simulink model "lab41"  (Simulink 8.0)
settings: Solver=ode45  StartTime=0.0  StopTime=10.0  RelTol=1e-3
undefined symbols (not defined in the file): get
libraries: commsequence2 x1, commseqgen2 x1, dspspect3 x1, simulink x1, commutil2 x1, dspsnks4 x1
settings Model: Creator=Dimav  LastModifiedBy=Dimav

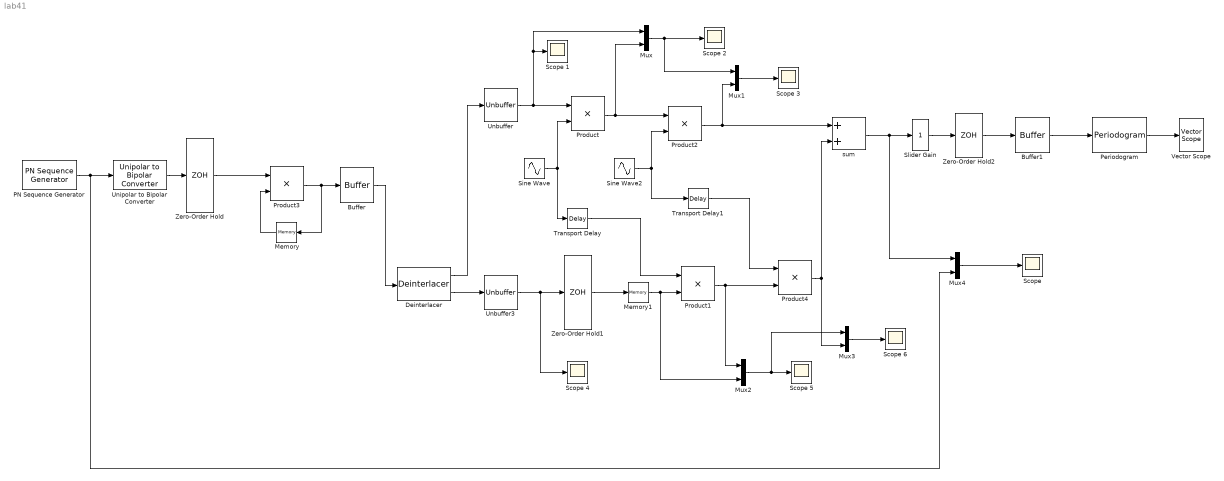
== system lab41 ==
  Buffer : Buffer  N=2  TreatMby1Signals=One channel
  Buffer1 : Buffer  TreatMby1Signals=One channel
  Deinterlacer : commsequence2/Deinterlacer
  Memory : Memory  X0=1  InheritSampleTime=on
  Memory1 : Memory  InheritSampleTime=on
  Mux{,1..4} (5 alike) : Mux  Inputs=2
  PN Sequence Generator : commseqgen2/PN Sequence Generator  poly=[1 0 0 0 0 1 1]  ini_sta=[0 0 0 0 0 1]  outBitMaskSource=Dialog parameter  shift=0  outVarSiz=off  maxOutSizeMode=Dialog parameter  maxOutSize=[10 1]  Ts=1/1200  frameBased=off  sampPerFrame=1  reset=off  bitPackedOutputs=off  outDataType=double  numPackedBits=8  bitPackDataSigned=off  bitPackedOutDType=double
  Periodogram : dspspect3/Periodogram  measurement=Power spectral density  wintype=Hamming  Rs=50  beta=5  winsamp=Symmetric  FFTImplementation=Auto  inheritFFT=off  fftsize=256  navg=4  inheritTs=on  Ts=1
  Product{,1..4} (5 alike) : Product  RndMeth=Zero
  Scope : Scope
      settings: SaveName=ScopeData6
  Scope {1..6} (6 alike) : Scope
      Scope 2 settings: SaveName=ScopeData2
      Scope 3 settings: SaveName=ScopeData3
      Scope 5 settings: SaveName=ScopeData4
      Scope 6 settings: SaveName=ScopeData5
  Sine Wave : Sin  Frequency=600*pi  Phase=-pi  SampleTime=0
  Sine Wave2 : Sin  Frequency=76000*pi  SampleTime=0
  Slider Gain : simulink/Math Operations/Slider Gain  low=0  gain=1  high=2
  Transport Delay : TransportDelay  DelayTime=1/1200
  Transport Delay1 : TransportDelay  DelayTime=3/38000/4
  Unbuffer : Unbuffer  SampleBasedProcessing=Same as frame based
  Unbuffer3 : Unbuffer  SampleBasedProcessing=Same as frame based
  Unipolar to Bipolar Converter : commutil2/Unipolar to Bipolar Converter  M=2  polarity=Positive  dataType=Inherit via internal rule
  Vector Scope : dspsnks4/Vector Scope  ScopeProperties=on  Domain=Time  HorizSpan=1  DisplayProperties=off  AxisGrid=on  Memory=off  FrameNumber=on  AxisLegend=off  AxisZoom=off  OpenScopeAtSimStart=on  OpenScopeImmediately=off  FigPos=get(0,'defaultfigureposition')  AxisProperties=off  XUnits=Hertz  XRange=[0...Fs/2]  InheritXIncr=on  XIncr=1  XLabel=Time  XLimit=Auto  XMin=0  XMax=1  XStart=0  YUnits=dB  YLabel=Amplitude  LineProperties=off  XAxisParamsVer=6.9
      settings: YMin=-10  YMax=10
  Zero-Order Hold : ZeroOrderHold  SampleTime=1/1200
  Zero-Order Hold1 : ZeroOrderHold  SampleTime=1/1200
  Zero-Order Hold2 : ZeroOrderHold  SampleTime=1/4000/3
  sum : Sum  Inputs=2  SaturateOnIntegerOverflow=on  InputSameDT=on  OutDataTypeStr=Inherit: Same as first input
  wires:
  Unipolar to Bipolar Converter/1 -> Zero-Order Hold/1
  Zero-Order Hold/1 -> Product3/1
  Memory/1 -> Product3/2
  Product3/1 -> Memory/1, Buffer/1
  Buffer/1 -> Deinterlacer/1
  Unbuffer/1 -> Mux/1, Scope 1/1, Product/1
  Sine Wave/1 -> Transport Delay/1, Product/2
  Unbuffer3/1 -> Scope 4/1, Zero-Order Hold1/1
  Zero-Order Hold1/1 -> Memory1/1
  Memory1/1 -> Mux2/2, Product1/2
  Transport Delay/1 -> Product1/1
  Product/1 -> Mux/2, Product2/1
  Sine Wave2/1 -> Transport Delay1/1, Product2/2
  Transport Delay1/1 -> Product4/1
  Product1/1 -> Mux2/1, Product4/2
  Mux/1 -> Mux1/1, Scope 2/1
  Mux1/1 -> Scope 3/1
  Product2/1 -> Mux1/2, sum/1
  Mux2/1 -> Mux3/1, Scope 5/1
  Mux3/1 -> Scope 6/1
  Product4/1 -> sum/2, Mux3/2
  PN Sequence Generator/1 -> Unipolar to Bipolar Converter/1, Mux4/2
  Mux4/1 -> Scope/1
  sum/1 -> Mux4/1, Slider Gain/1
  Slider Gain/1 -> Zero-Order Hold2/1
  Zero-Order Hold2/1 -> Buffer1/1
  Buffer1/1 -> Periodogram/1
  Periodogram/1 -> Vector Scope/1
  Deinterlacer/1 -> Unbuffer/1
  Deinterlacer/2 -> Unbuffer3/1
